simulink model "mchecksum_coverage"  (Simulink 6.1)
settings: Solver=FixedStepDiscrete  StartTime=0.0  StopTime=10.0  FixedStep=1  RelTol=1e-3
libraries: mchecksum_coverage_lib x2
settings Model: Creator=mshakeri  LastModifiedBy=mshakeri  ExtModeAutoUpdateStatusClock=off  StrictBusMsg=ErrorLevel1
settings OptimizationCC: InlineInvariantSignals=off
settings DebuggingCC: SolverPrmCheckMsg=warning

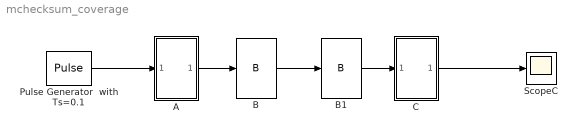
== system mchecksum_coverage ==
  A : Subsystem  TreatAsAtomicUnit=on
  B : mchecksum_coverage_lib/B
  B1 : mchecksum_coverage_lib/B
  C : Subsystem  TreatAsAtomicUnit=on
  Pulse Generator  with Ts=0.1 : DiscretePulseGenerator
  ScopeC : Scope
      settings: TimeRange=10  YMin=0  YMax=15  SaveName=ScopeDataC  DataFormat=Array
  wires:
  Pulse Generator  with Ts=0.1/1 -> A/1(In1)
  C/1(Out1) -> ScopeC/1
  A/1(Out1) -> B/1
  B/1 -> B1/1
  B1/1 -> C/1(In1)

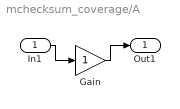
== system mchecksum_coverage/A ==
  In1 : Inport  Port=1  LatchInput=off
  Gain : Gain
  Out1 : Outport
  wires:
  In1/1 -> Gain/1
  Gain/1 -> Out1/1

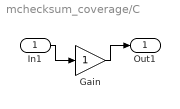
== system mchecksum_coverage/C ==
  In1 : Inport  Port=1  LatchInput=off
  Gain : Gain
  Out1 : Outport
  wires:
  Gain/1 -> Out1/1
  In1/1 -> Gain/1
